simulink model "Identify_model_right_R2015a"  (R2015a)
settings: Solver=ode45  StartTime=0.0  StopTime=147  RelTol=1e-3
values from neighbouring files (symbols this model uses):
  a0 = (pi^2/k_max^2) + (a1^2/4)    [Identify_right.m]
  a1 = -(1/k_max)*2*log((y_max/y0)-1)    [Identify_right.m]
  b0 = a0*y0/r    [Identify_right.m]
  r = wheel_diameter*pi*(100/60)    (= 2.0276362585)    [Identify_right.m]
  sample_time = 1    [Identify_right.m]
settings Model: CovModelRefEnable=off  Creator=ryodo  LastModifiedBy=ryodo
settings DataIOCC: SaveFormat=Dataset
settings HardwareCC: ProdBitPerPointer=64  ProdLargestAtomicFloat=Float  ProdIntDivRoundTo=Zero  ProdEndianess=LittleEndian  ProdHWDeviceType=Specified
settings GRTTargetCC: GeneratePreprocessorConditionals=Use local settings

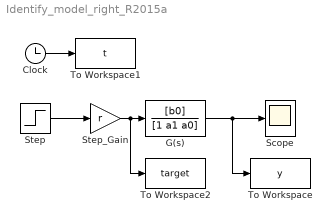
== system Identify_model_right_R2015a ==
  Clock : Clock
  G(s) : TransferFcn  Numerator=[b0]  Denominator=[1 a1 a0]
  Scope : Scope
      settings: TimeRange=auto  MaxDataPoints=5000  SaveToWorkspace=off  SaveName=ScopeData  YMin=-0.30837  YMax=2.77533  SampleTime=-1
  Step : Step  Time=0  SampleTime=sample_time
  Step_Gain : Gain  Gain=r
  To Workspace : ToWorkspace  VariableName=y  SampleTime=sample_time
  To Workspace1 : ToWorkspace  VariableName=t  SampleTime=sample_time
  To Workspace2 : ToWorkspace  VariableName=target  SampleTime=sample_time
  wires:
  Step_Gain/1 -> To Workspace2/1, G(s)/1
  Step/1 -> Step_Gain/1
  G(s)/1 -> Scope/1, To Workspace/1
  Clock/1 -> To Workspace1/1
